simulink model "AirbrakesPhysics"  (R2025b)
settings: Solver=VariableStepAuto  StartTime=0.0  StopTime=30  RelTol=1e-3
libraries: aerolibatmos2 x1, slpidlib x1
settings Model: Creator=Bingc  LastModifiedBy=Bingc

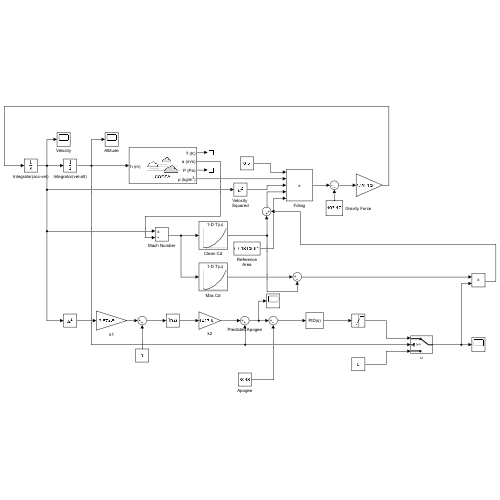
[thumbnail: Simulink's stored preview of the top-level diagram]
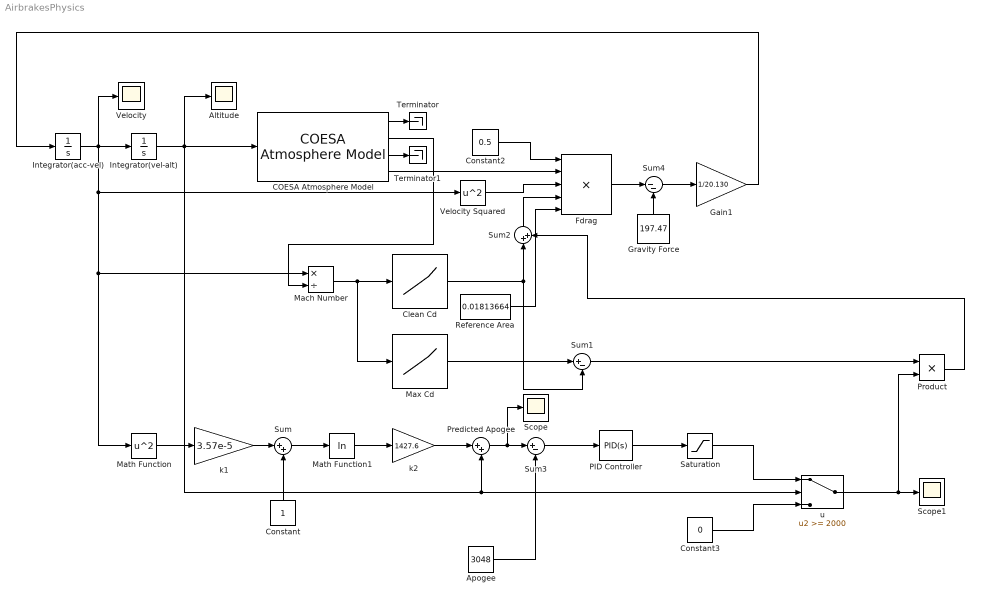
== system AirbrakesPhysics ==
  Altitude : Scope
      settings: ActiveDisplayYMinimum=2007.91841246052  ActiveDisplayYMaximum=5522.6732853303711
  Apogee : Constant  Value=3048
  COESA Atmosphere Model : aerolibatmos2/COESA Atmosphere Model  units=Metric (MKS)  spec=1976 COESA-extended U.S. Standard Atmosphere  model=Profile  profile_var=High temperature  profile_percent=1%  profile_alt=5 km (16404 ft)  envelope_var=High temperature  envelope_percent=1%  action=Warning
  Clean Cd : Lookup_n-D  NumberOfTableDimensions=1  BreakpointsForDimension1=[0.1, 0.2, 0.3, 0.4, 0.5, 0.6, 0.7, 0.8, 0.9]  Table=[0.384, 0.38, 0.387, 0.398, 0.411, 0.429, 0.451, 0.48, 0.528]  InternalRulePriority=Speed  RndMeth=Simplest
  Constant : Constant
  Constant2 : Constant  Value=0.5
  Constant3 : Constant  Value=0
  Fdrag : Product  Inputs=5
  Gain1 : Gain  Gain=1/20.130
  Gravity Force : Constant  Value=197.47
  Integrator(acc-vel) : Integrator  InitialCondition=298.3
  Integrator(vel-alt) : Integrator  InitialCondition=807.72
  Mach Number : Product  Inputs=*/
  Math Function : Math  Operator=square
  Math Function1 : Math  Operator=log
  Max Cd : Lookup_n-D  NumberOfTableDimensions=1  BreakpointsForDimension1=[0.1, 0.2, 0.3, 0.4, 0.5, 0.6, 0.7, 0.8, 0.9]  Table=[1.484, 1.48, 1.487, 1.498, 1.511, 1.529, 1.551, 1.58, 1.628]  InternalRulePriority=Speed  RndMeth=Simplest
  PID Controller : slpidlib/PID Controller  Controller=PID  Form=Parallel  TimeDomain=Continuous-time  UseExternalTs=off  SampleTime=-1  IntegratorMethod=Forward Euler  FilterMethod=Forward Euler  ControllerParametersSource=internal  P=-0.01  I=1  UseKiTs=off  D=-0.05  UseExternalDerivativeSource=off  N=100  UseFilter=on  TunerSelectOption=Transfer Function Based (PID Tuner App)  InitialConditionSource=internal  InitialConditionForIntegrator=0  InitialConditionForFilter=0  DifferentiatorICPrevScaledInput=0  ExternalReset=none  TrackingMode=off  Kt=1  LimitOutput=off  SatLimitsSource=internal  UpperSaturationLimit=inf  LowerSaturationLimit=-inf  LinearizeAsGain=on  AntiWindupMode=none  Kb=1  LimitIntegrator=off  UpperIntegratorSaturationLimit=inf  LowerIntegratorSaturationLimit=-inf  POutMin=[]  POutMax=[]  IOutMin=[]  IOutMax=[]  DOutMin=[]  DOutMax=[]  NOutMin=[]  NOutMax=[]  SumOutMin=[]  SumOutMax=[]  SaturationOutMin=[]  SaturationOutMax=[]  PParamMin=[]  PParamMax=[]  IParamMin=[]  IParamMax=[]  DParamMin=[]  DParamMax=[]  NParamMin=[]  NParamMax=[]  KbParamMin=[]  KbParamMax=[]  KtParamMin=[]  KtParamMax=[]  KbOutMin=[]  KbOutMax=[]  KtOutMin=[]  KtOutMax=[]  IntegratorOutMin=[]  IntegratorOutMax=[]  FilterOutMin=[]  FilterOutMax=[]  SumI1OutMin=[]  SumI1OutMax=[]  SumI2OutMin=[]  SumI2OutMax=[]  SumI3OutMin=[]  SumI3OutMax=[]  SumI4OutMin=[]  SumI4OutMax=[]  SumDOutMin=[]  SumDOutMax=[]  DifferentiatorOutMin=[]  DifferentiatorOutMax=[]  FilterDiffOutCoefMin=[]  FilterDiffOutCoefMax=[]  ReciprocalOutMin=[]  ReciprocalOutMax=[]  SumDenOutMin=[]  SumDenOutMax=[]  SumNumOutMin=[]  SumNumOutMax=[]  DivideOutMin=[]  DivideOutMax=[]  UdiffTsProdOutMin=[]  UdiffTsProdOutMax=[]  NTsProdOutMin=[]  NTsProdOutMax=[]  UintegralTsProdOutMin=[]  UintegralTsProdOutMax=[]  UngainTsProdOutMin=[]  UngainTsProdOutMax=[]  ClampingZeroOutDataTypeStr=Inherit: Inherit via back propagation  ClampingZeroOutMin=[]  ClampingZeroOutMax=[]  FilterDenConstantOutDataTypeStr=Inherit: Inherit via back propagation  FilterDenConstantOutMin=[]  FilterDenConstantOutMax=[]  PCopyOutDataTypeStr=Inherit: Inherit via back propagation  PCopyOutMin=[]  PCopyOutMax=[]  NCopyOutDataTypeStr=Inherit: Inherit via back propagation  NCopyOutMin=[]  NCopyOutMax=[]  IntegratorContinuousStateAttributes=''  IntegratorStateMustResolveToSignalObject=off  IntegratorRTWStateStorageClass=Auto  FilterContinuousStateAttributes=''  FilterStateMustResolveToSignalObject=off  FilterRTWStateStorageClass=Auto  ParallelPVariant=InternalParameters  IdealPVariant=Disabled  IVariant=InternalParameters  DVariant=InternalParameters  IntegratorVariant=Continuous  SatVariant=Disabled  AWVariant=Passthrough  PCopyVariant=Disabled  TRVariant=Disabled  FdbkBlocksVariant=Forward  IdealPFdbkVariant=Disabled  SatFdbkVariant=Disabled  DerivativeFilterVariant=ContFilter  NVariant=InternalParameters  NCopyVariant=Disabled  FilterICVariant=InternalICsFilter  IntegratorICVariant=InternalICs  ExternalResetVariant=Disabled  TRSumVariant=Passthrough  SumFdbkVariant=Disabled  SumVariant=Sum_PID  TsampFilterVariant=InternalTs  TsampNgainVariant=Passthrough  TsampIntegralVariant=Disabled_SignalSpec  ExternalSaturationOutDataTypeStr=Inherit: Same as second input  DerivativeSourceVariant=ErrorSignal  PreIntVariant=InternalPreInt
  Predicted Apogee : Sum  Inputs=|++
  Product : Product
  Reference Area : Constant  Value=0.01813664
  Saturation : Saturate  UpperLimit=1  LowerLimit=0
  Scope : Scope
      settings: ActiveDisplayYMinimum=2032.3579901363989  ActiveDisplayYMaximum=4026.7845518006293  DataLoggingVariableName=ScopeData2
  Scope1 : Scope
      settings: ActiveDisplayYMinimum=-0.12499999999999997  ActiveDisplayYMaximum=1.125  DataLoggingVariableName=ScopeData3
  Sum : Sum  Inputs=|++
  Sum1 : Sum  Inputs=|+-
  Sum2 : Sum  Inputs=|++
  Sum3 : Sum  Inputs=|+-
  Sum4 : Sum  Inputs=|--
  Terminator : Terminator
  Terminator1 : Terminator
  Velocity : Scope
      settings: ActiveDisplayYMinimum=-1  ActiveDisplayYMaximum=1
  Velocity Squared : Math  Operator=square
  k1 : Gain  Gain=3.57e-5
  k2 : Gain  Gain=1427.6
  u : Switch  Threshold=2000  SaturateOnIntegerOverflow=off  InputSameDT=off
  wires:
  Clean Cd/1 -> Sum2/1, Sum1/2
  Integrator(vel-alt)/1 -> COESA Atmosphere Model/1, Predicted Apogee/2, u/2, Altitude/1
  COESA Atmosphere Model/4 -> Fdrag/2
  Integrator(acc-vel)/1 -> Velocity Squared/1, Math Function/1, Mach Number/1, Integrator(vel-alt)/1, Velocity/1
  Sum4/1 -> Gain1/1
  Gravity Force/1 -> Sum4/2
  Mach Number/1 -> Max Cd/1, Clean Cd/1
  COESA Atmosphere Model/2 -> Mach Number/2
  Constant2/1 -> Fdrag/1
  Reference Area/1 -> Fdrag/5
  Gain1/1 -> Integrator(acc-vel)/1
  Fdrag/1 -> Sum4/1
  Velocity Squared/1 -> Fdrag/3
  COESA Atmosphere Model/1 -> Terminator/1
  COESA Atmosphere Model/3 -> Terminator1/1
  Max Cd/1 -> Sum1/1
  Sum1/1 -> Product/1
  u/1 -> Product/2, Scope1/1
  Product/1 -> Sum2/2
  Sum2/1 -> Fdrag/4
  Math Function/1 -> k1/1
  k1/1 -> Sum/1
  Constant/1 -> Sum/2
  Math Function1/1 -> k2/1
  k2/1 -> Predicted Apogee/1
  Sum/1 -> Math Function1/1
  Predicted Apogee/1 -> Scope/1, Sum3/1
  Apogee/1 -> Sum3/2
  Sum3/1 -> PID Controller/1
  PID Controller/1 -> Saturation/1
  Saturation/1 -> u/1
  Constant3/1 -> u/3
